simulink model "Temporal2"  (R2020b)
settings: Solver=FixedStepDiscrete  StartTime=0.0  StopTime=20  FixedStep=0.1  RelTol=1e-3  EnableMultiTasking=on
settings Model: Creator=bzhan  LastModifiedBy=apple
settings SolverCC: AutoInsertRateTranBlk=on
settings DataIOCC: LimitDataPoints=on
settings OptimizationCC: LifeSpan=inf
settings DebuggingCC: AllowSymbolicDim=off  SFUnexpectedBacktrackingDiag=warning  SFNoUnconditionalDefaultTransitionDiag=warning  SFExecutionAtInitializationDiag=none  ArithmeticOperatorsInVariantConditions=warning
settings SFSimCC: SimUseLocalCustomCode=off  CustomCodeUndefinedFunction=UseInterfaceOnly
settings RTWCC: RTWUseLocalCustomCode=off
settings CodeAppCC: StateflowObjectComments=on
settings GRTTargetCC: TargetLangStandard=C89/C90 (ANSI)
settings ConfigComp: CovMetricSettings=dw  CovSaveCumulativeToWorkspaceVar=on  CovSaveSingleToWorkspaceVar=on  CovExternalEMLEnable=off  CovSFcnEnable=off

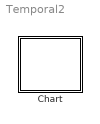
== system Temporal2 ==
  Chart : Stateflow chart  TreatAsAtomicUnit=on

== stateflow chart Temporal2/Chart ==
  settings: updateMethod=DISCRETE  sampleTime=1
  state A
    en: f("en_A"); ra=2;
  state B
    en: f("en_B"); rb=3;
  (default) -> A
  A -> B : after(ra,sec)
  B -> A : after(rb,sec)
  data: s function_input; ra local; rb local
  function f(s):
    | function f(s)
    |   fprintf(s+"\n");
